simulink model "process_test"  (R2017b)
settings: Solver=ode45  StartTime=0.0  StopTime=1000  RelTol=1e-3  EnableMultiTasking=on
libraries: simulink x10
settings Model: Creator=bl405  LastModifiedBy=Bailey Brookes
settings DataIOCC: ExternalInput=[0 2]  InitialState=[]  LimitDataPoints=on  LoadExternalInput=on  LoadInitialState=on  SaveFormat=Array
settings OptimizationCC: DefaultParameterBehavior=Inlined  BufferReuse=off  LifeSpan=inf
settings DebuggingCC: InitInArrayFormatMsg=none  SFUnexpectedBacktrackingDiag=warning  SFNoUnconditionalDefaultTransitionDiag=warning  SFExecutionAtInitializationDiag=none
settings HardwareCC: ProdBitPerPointer=32  ProdBitPerSizeT=32  ProdBitPerPtrDiffT=32  ProdLargestAtomicFloat=None  ProdIntDivRoundTo=Undefined  ProdEndianess=Unspecified  ProdWordSize=32  ProdHWDeviceType=32-bit Generic
settings ModelReferenceCC: PropagateSignalLabelsOutOfModel=off
settings CodeAppCC: StateflowObjectComments=on
settings GRTTargetCC: TargetLangStandard=C89/C90 (ANSI)  GeneratePreprocessorConditionals=Disable all
settings ConfigComp: CovMetricSettings=dw  CovHtmlReporting=on  CovSaveCumulativeToWorkspaceVar=on  CovSaveSingleToWorkspaceVar=on  CovExternalEMLEnable=off

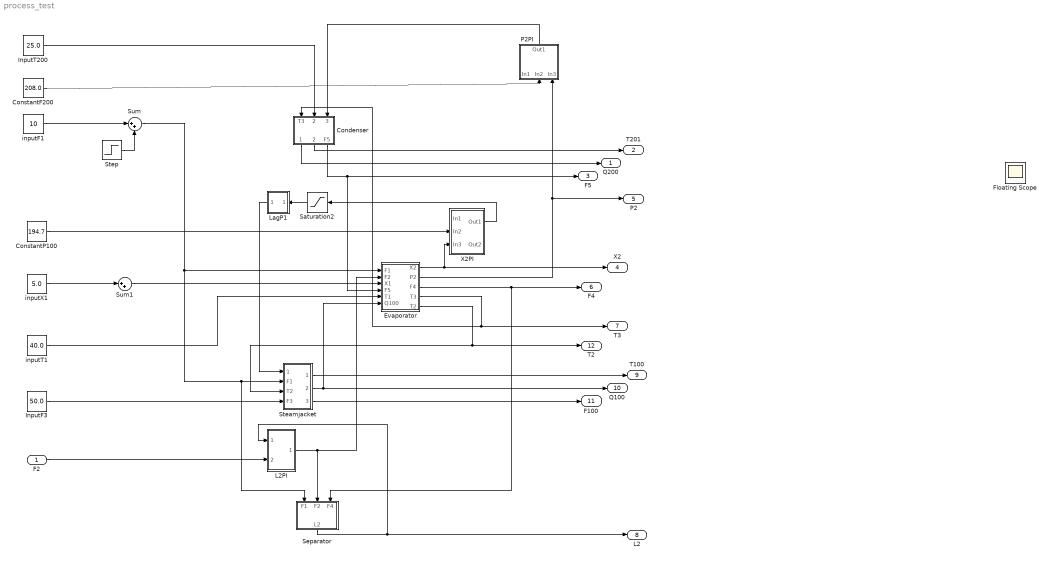
== system process_test ==
  F2 : Inport
  Condenser : Subsystem
  ConstantF200 : Constant  Value=208.0
  ConstantP100 : Constant  Value=194.7
  Evaporator : Subsystem
  Floating Scope : Scope
      settings: Floating=on
  InputF3 : Constant  Value=50.0
  "InputT200 " : Constant  Value=25.0
  L2PI : Subsystem
  LagP1 : Subsystem
  P2PI : Subsystem
  Saturation2 : Saturate  UpperLimit=194.7*2  LowerLimit=0
  Separator : Subsystem
  Steamjacket : Subsystem
  Step : Step  After=20  SampleTime=0
  Sum : Sum  Inputs=|++
  Sum1 : Sum  Inputs=|++
  X2PI : Subsystem
  inputF1 : Constant  Value=10
  inputT1 : Constant  Value=40.0
  inputX1 : Constant  Value=5.0
  Q200 : Outport
  T201 : Outport  Port=2
  F5 : Outport  Port=3
  X2 : Outport  Port=4
  P2 : Outport  Port=5
  F4 : Outport  Port=6
  T3 : Outport  Port=7
  L2 : Outport  Port=8
  T100 : Outport  Port=9
  Q100 : Outport  Port=10
  F100 : Outport  Port=11
  T2 : Outport  Port=12
  wires:
  Evaporator/4(T3) -> T3/1, Condenser/1(T3)
  "InputT200 "/1 -> Condenser/2(T200)
  Condenser/1(Q200) -> Q200/1
  Condenser/2(T201) -> T201/1
  Sum1/1 -> Evaporator/3(X1)
  Condenser/3(F5) -> F5/1, Evaporator/4(F5)
  Steamjacket/2(Q100) -> Evaporator/6(Q100), Q100/1
  Evaporator/3(F4) -> F4/1, Separator/3(F4)
  Sum/1 -> Evaporator/1("F1 "), Separator/1(F1), Steamjacket/2(F1)
  Evaporator/5(T2) -> Steamjacket/3(T2), T2/1
  InputF3/1 -> Steamjacket/4(F3)
  Steamjacket/1(T100) -> T100/1
  Steamjacket/3(F100) -> F100/1
  inputT1/1 -> Evaporator/5(T1)
  Separator/1(L2) -> L2PI/1(In1), L2/1
  L2PI/1(Out1) -> Evaporator/2("F2 "), Separator/2(F2)
  LagP1/1(output) -> Steamjacket/1(P100)
  inputF1/1 -> Sum/1
  inputX1/1 -> Sum1/1
  F2/1 -> L2PI/2(Inport F2)
  Step/1 -> Sum/2
  Saturation2/1 -> LagP1/1(Input)
  Evaporator/1(X2) -> X2/1, X2PI/3(In3)
  ConstantP100/1 -> X2PI/2(In2)
  X2PI/1(Out1) -> Saturation2/1
  Evaporator/2(P2) -> P2PI/3(In3), P2/1
  ConstantF200/1 -> P2PI/2(In2)
  P2PI/1(Out1) -> Condenser/3(F200)

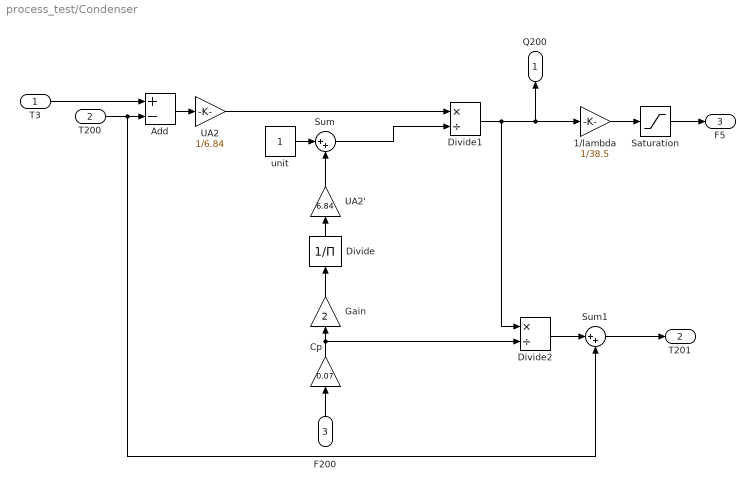
== system process_test/Condenser ==
  T3 : Inport
  T200 : Inport  Port=2
  F200 : Inport  Port=3
  1/lambda : Gain  Gain=1/38.5
  Add : Sum  Inputs=+-
  Cp : Gain  Gain=0.07
  Divide : Product  Inputs=/
  Divide1 : Product  Inputs=*/
  Divide2 : Product  Inputs=*/
  Gain : Gain  Gain=2
  Saturation : Saturate  UpperLimit=16  LowerLimit=0
  Sum : Sum  Inputs=|++
  Sum1 : Sum  Inputs=|++
  UA2 : Gain  Gain=1/6.84
  UA2' : Gain  Gain=6.84
  unit : Constant
  Q200 : Outport
  T201 : Outport  Port=2
  F5 : Outport  Port=3
  wires:
  T200/1 -> Add/2, Sum1/2
  Gain/1 -> Divide/1
  UA2/1 -> Divide1/1
  Divide2/1 -> Sum1/1
  Divide1/1 -> Q200/1, 1/lambda/1, Divide2/1
  Add/1 -> UA2/1
  UA2'/1 -> Sum/2
  unit/1 -> Sum/1
  Divide/1 -> UA2'/1
  Cp/1 -> Gain/1, Divide2/2
  T3/1 -> Add/1
  Sum1/1 -> T201/1
  Sum/1 -> Divide1/2
  F200/1 -> Cp/1
  1/lambda/1 -> Saturation/1
  Saturation/1 -> F5/1

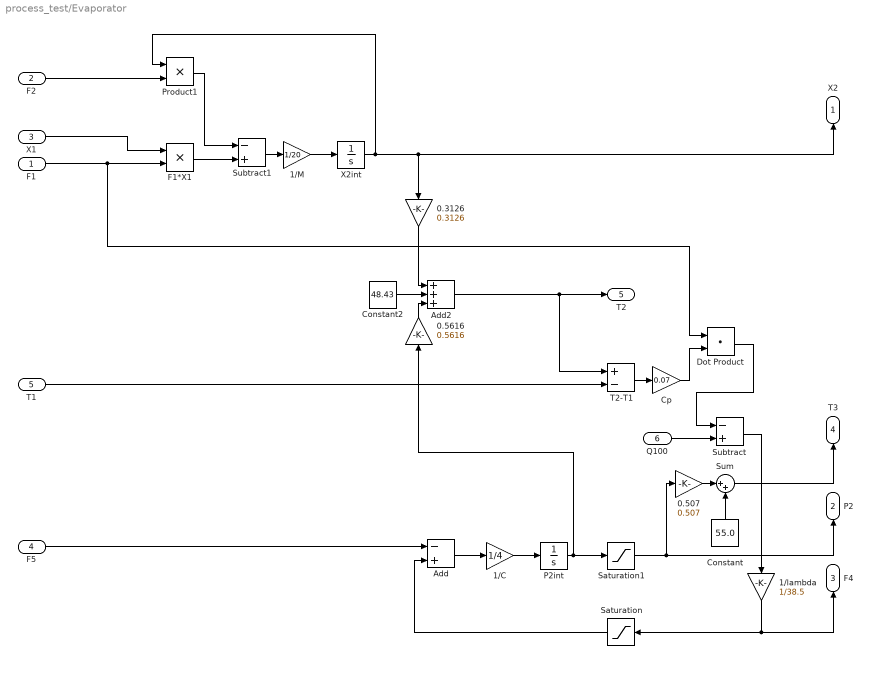
== system process_test/Evaporator ==
  "F1 " : Inport
  "F2 " : Inport  Port=2
  X1 : Inport  Port=3
  F5 : Inport  Port=4
  T1 : Inport  Port=5
  Q100 : Inport  Port=6
  0.3126 : Gain  Gain=0.3126
  0.507 : Gain  Gain=0.507
  0.5616 : Gain  Gain=0.5616
  1/C : Gain  Gain=1/4
  1/M : Gain  Gain=1/20
  1/lambda : Gain  Gain=1/38.5
  Add : Sum  Inputs=-+
  Add2 : Sum  Inputs=+++
  Constant : Constant  Value=55.0
  Constant2 : Constant  Value=48.43
  Cp : Gain  Gain=0.07
  Dot Product : DotProduct  InputSameDT=on  OutDataTypeStr=Inherit: Inherit via internal rule
  F1*X1 : Product
  P2int : Integrator  InitialCondition=50.5
  Product1 : Product
  Saturation : Saturate  UpperLimit=16  LowerLimit=0
  Saturation1 : Saturate  UpperLimit=110.0  LowerLimit=0
  Subtract : Sum  Inputs=-+
  Subtract1 : Sum  Inputs=-+
  Sum : Sum  Inputs=|++
  T2-T1 : Sum  Inputs=+-
  X2int : Integrator  InitialCondition=25.0
  X2 : Outport
  P2 : Outport  Port=2
  F4 : Outport  Port=3
  T3 : Outport  Port=4
  T2 : Outport  Port=5
  wires:
  Product1/1 -> Subtract1/1
  "F2 "/1 -> Product1/2
  P2int/1 -> 0.5616/1, Saturation1/1
  "F1 "/1 -> F1*X1/2, Dot Product/1
  Q100/1 -> Subtract/2
  Sum/1 -> T3/1
  Constant2/1 -> Add2/2
  0.3126/1 -> Add2/1
  0.5616/1 -> Add2/3
  Constant/1 -> Sum/2
  Cp/1 -> Dot Product/2
  Add/1 -> 1/C/1
  Add2/1 -> T2/1, T2-T1/1
  1/M/1 -> X2int/1
  F5/1 -> Add/1
  Subtract1/1 -> 1/M/1
  T1/1 -> T2-T1/2
  1/lambda/1 -> Saturation/1, F4/1
  Subtract/1 -> 1/lambda/1
  F1*X1/1 -> Subtract1/2
  0.507/1 -> Sum/1
  Dot Product/1 -> Subtract/1
  1/C/1 -> P2int/1
  X2int/1 -> X2/1, 0.3126/1, Product1/1
  X1/1 -> F1*X1/1
  T2-T1/1 -> Cp/1
  Saturation/1 -> Add/2
  Saturation1/1 -> 0.507/1, P2/1

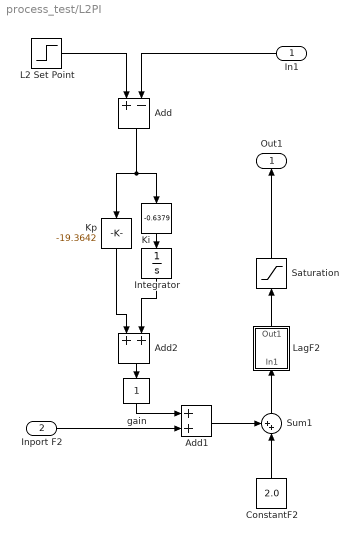
== system process_test/L2PI ==
  In1 : Inport
  Inport F2 : Inport  Port=2
  Add : Sum  Inputs=+-
  Add1 : Sum
  Add2 : Sum
  ConstantF2 : Constant  Value=2.0
  Integrator : Integrator
  Ki : simulink/Math Operations/Slider Gain  gain=-0.6379  low=-140  high=20
  Kp : simulink/Math Operations/Slider Gain  gain=-19.3642  low=-169.8244  high=0
  L2 Set Point : Step  Before=1  After=1.  SampleTime=0
  LagF2 : Subsystem
  Saturation : Saturate  UpperLimit=4.0  LowerLimit=0
  Sum1 : Sum  Inputs=++|
  gain : simulink/Math Operations/Slider Gain  gain=1  low=-140  high=1
  Out1 : Outport
  wires:
  Ki/1 -> Integrator/1
  LagF2/1(Out1) -> Saturation/1
  Kp/1 -> Add2/1
  Sum1/1 -> LagF2/1(In1)
  Inport F2/1 -> Add1/2
  L2 Set Point/1 -> Add/1
  Saturation/1 -> Out1/1
  Add1/1 -> Sum1/1
  ConstantF2/1 -> Sum1/2
  Add/1 -> Ki/1, Kp/1
  Integrator/1 -> Add2/2
  Add2/1 -> gain/1
  In1/1 -> Add/2
  gain/1 -> Add1/1

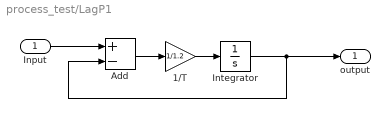
== system process_test/LagP1 ==
  Input : Inport
  1/T : Gain  Gain=1/1.2
  Add : Sum  Inputs=+-
  Integrator : Integrator  InitialCondition=194.7
  output : Outport
  wires:
  Input/1 -> Add/1
  Add/1 -> 1/T/1
  1/T/1 -> Integrator/1
  Integrator/1 -> Add/2, output/1

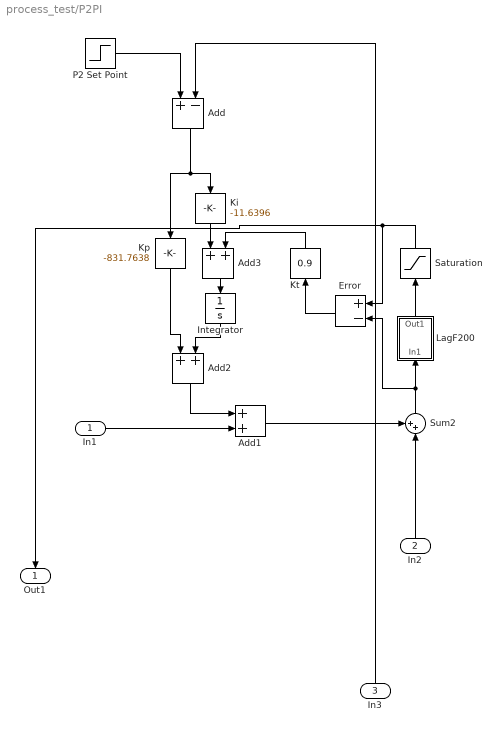
== system process_test/P2PI ==
  In1 : Inport
  In2 : Inport  Port=2
  In3 : Inport  Port=3
  Add : Sum  Inputs=+-
  Add1 : Sum
  Add2 : Sum
  Add3 : Sum
  Error : Sum  Inputs=+-
  Integrator : Integrator
  Ki : simulink/Math Operations/Slider Gain  gain=-11.6396  low=-140  high=20
  Kp : simulink/Math Operations/Slider Gain  gain=-831.7638  low=-831.7638  high=831.7638
  Kt : simulink/Math Operations/Slider Gain  gain=0.9  low=-831.7638  high=831.7638
  LagF200 : Subsystem
  P2 Set Point : Step  Before=50.5  After=50.5  SampleTime=0
  Saturation : Saturate  UpperLimit=416  LowerLimit=0
  Sum2 : Sum  Inputs=++|
  Out1 : Outport
  wires:
  In3/1 -> Add/2
  Kt/1 -> Add3/2
  Add3/1 -> Integrator/1
  Ki/1 -> Add3/1
  LagF200/1(Out1) -> Saturation/1
  Kp/1 -> Add2/1
  Sum2/1 -> Error/2, LagF200/1(In1)
  In1/1 -> Add1/2
  P2 Set Point/1 -> Add/1
  Add1/1 -> Sum2/1
  In2/1 -> Sum2/2
  Add/1 -> Ki/1, Kp/1
  Integrator/1 -> Add2/2
  Add2/1 -> Add1/1
  Saturation/1 -> Out1/1, Error/1
  Error/1 -> Kt/1

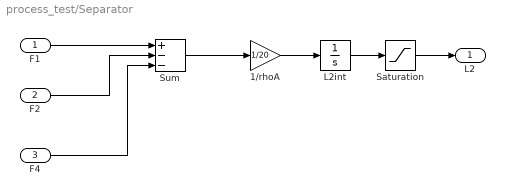
== system process_test/Separator ==
  F1 : Inport
  F2 : Inport  Port=2
  F4 : Inport  Port=3
  1/rhoA : Gain  Gain=1/20
  L2int : Integrator  InitialCondition=1
  Saturation : Saturate  UpperLimit=2  LowerLimit=0
  Sum : Sum  Inputs=+--
  L2 : Outport
  wires:
  F4/1 -> Sum/3
  Sum/1 -> 1/rhoA/1
  F1/1 -> Sum/1
  F2/1 -> Sum/2
  1/rhoA/1 -> L2int/1
  L2int/1 -> Saturation/1
  Saturation/1 -> L2/1

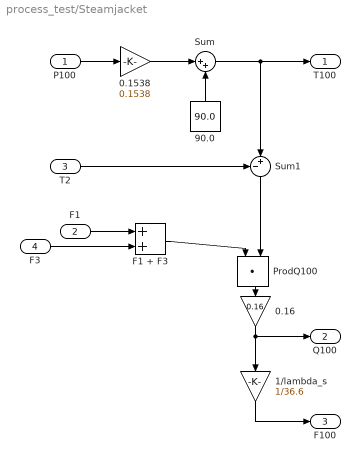
== system process_test/Steamjacket ==
  P100 : Inport
  F1 : Inport  Port=2
  T2 : Inport  Port=3
  F3 : Inport  Port=4
  0.1538 : Gain  Gain=0.1538
  0.16 : Gain  Gain=0.16
  1/lambda_s : Gain  Gain=1/36.6
  90.0 : Constant  Value=90.0
  F1 + F3 : Sum
  ProdQ100 : DotProduct  InputSameDT=on  OutDataTypeStr=Inherit: Inherit via internal rule
  Sum : Sum  Inputs=|++
  Sum1 : Sum  Inputs=-+|
  T100 : Outport
  Q100 : Outport  Port=2
  F100 : Outport  Port=3
  wires:
  F1/1 -> F1 + F3/1
  F1 + F3/1 -> ProdQ100/1
  Sum1/1 -> ProdQ100/2
  1/lambda_s/1 -> F100/1
  T2/1 -> Sum1/1
  P100/1 -> 0.1538/1
  F3/1 -> F1 + F3/2
  ProdQ100/1 -> 0.16/1
  0.16/1 -> Q100/1, 1/lambda_s/1
  90.0/1 -> Sum/2
  0.1538/1 -> Sum/1
  Sum/1 -> T100/1, Sum1/2

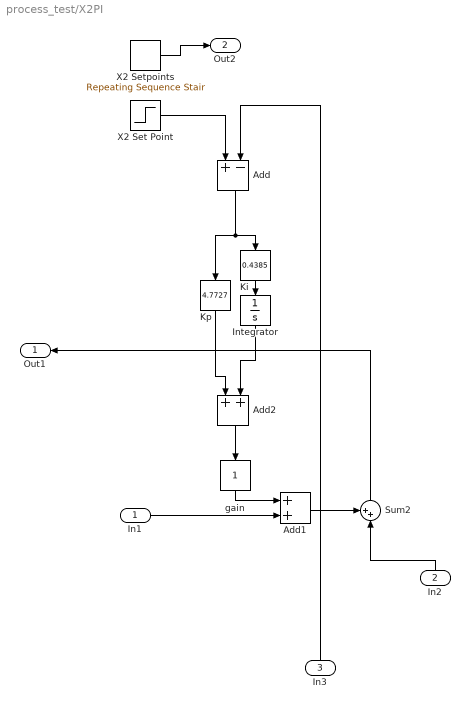
== system process_test/X2PI ==
  In1 : Inport
  In2 : Inport  Port=2
  In3 : Inport  Port=3
  Add : Sum  Inputs=+-
  Add1 : Sum
  Add2 : Sum
  Integrator : Integrator
  Ki : simulink/Math Operations/Slider Gain  gain=0.4385  low=-140  high=20
  Kp : simulink/Math Operations/Slider Gain  gain=4.7727  low=-831.7638  high=20
  Sum2 : Sum  Inputs=++|
  X2 Set Point : Step  Before=25.0  After=25.0  SampleTime=0
  X2 Setpoints : simulink/Sources/Repeating Sequence Stair  OutValues=[25:35 35:-1:15 15 15 15 35 35 35 35 15 15 15 25 25 25 25 25 25 25 25 25 25 25 ].'  tsamp=100  OutMin=[]  OutMax=[]  OutDataTypeStr=double  OutputDataTypeScalingMode=double  OutDataType=fixdt(0,8)  ConRadixGroup=Best Precision: Vector-wise  OutScaling=2^-12
  gain : simulink/Math Operations/Slider Gain  gain=1  low=-831.7638  high=20
  Out1 : Outport
  Out2 : Outport  Port=2
  wires:
  In3/1 -> Add/2
  Ki/1 -> Integrator/1
  Kp/1 -> Add2/1
  In1/1 -> Add1/2
  X2 Set Point/1 -> Add/1
  Add1/1 -> Sum2/1
  In2/1 -> Sum2/2
  Add/1 -> Ki/1, Kp/1
  Integrator/1 -> Add2/2
  Add2/1 -> gain/1
  gain/1 -> Add1/1
  Sum2/1 -> Out1/1
  X2 Setpoints/1 -> Out2/1

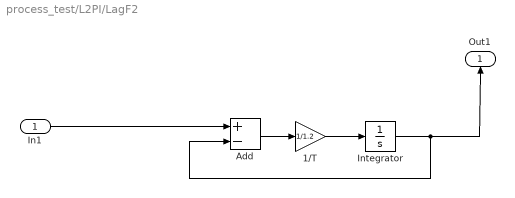
== system process_test/L2PI/LagF2 ==
  In1 : Inport
  1/T : Gain  Gain=1/1.2
  Add : Sum  Inputs=+-
  Integrator : Integrator  InitialCondition=2.0
  Out1 : Outport
  wires:
  1/T/1 -> Integrator/1
  Add/1 -> 1/T/1
  In1/1 -> Add/1
  Integrator/1 -> Out1/1, Add/2

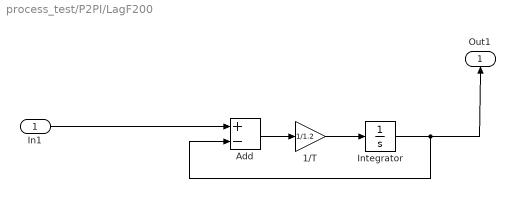
== system process_test/P2PI/LagF200 ==
  In1 : Inport
  1/T : Gain  Gain=1/1.2
  Add : Sum  Inputs=+-
  Integrator : Integrator  InitialCondition=208.0
  Out1 : Outport
  wires:
  1/T/1 -> Integrator/1
  Add/1 -> 1/T/1
  In1/1 -> Add/1
  Integrator/1 -> Out1/1, Add/2
